simulink model "Delfin"  (R2018b)
settings: Solver=VariableStepAuto  StartTime=0.0  StopTime=0.2  RelTol=1e-3
undefined symbols (not defined in the file): fn, L1b, R1b, Stv, U1, U2, Ukz
libraries: powerlib x34, peRmsMeasurement x10, powerlib_meascontrol x2
settings Model: Creator=sr1  LastModifiedBy=sr1

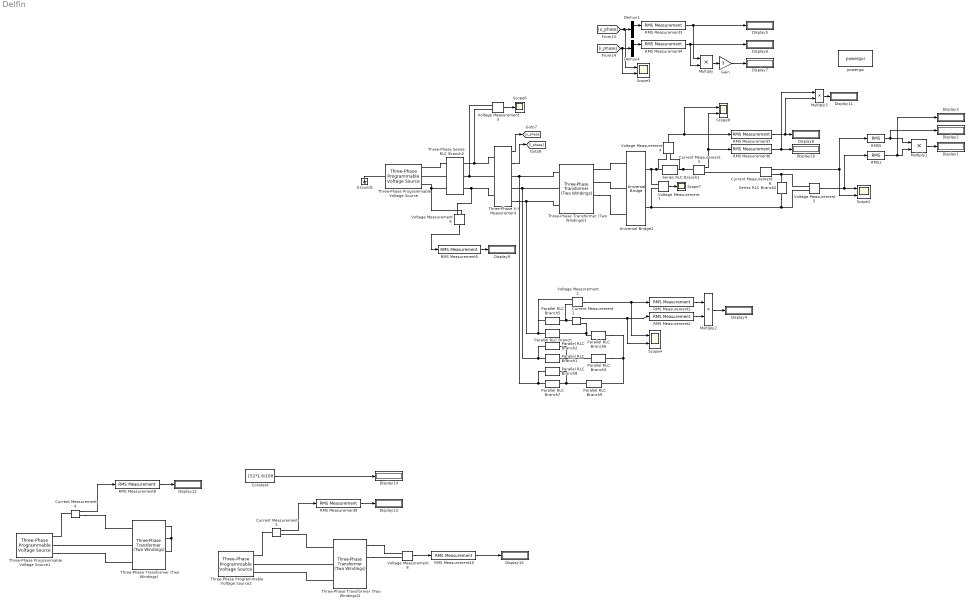
== system Delfin ==
  Constant : Constant  Value=152*1.6/100
  Current Measurement{1,3..6} (5 alike) : powerlib/Measurements/Current Measurement  PhasorSimulation=off  OutputType=Complex  PSBequivalent=0
  Demux1 : Demux  Outputs=3
  Demux4 : Demux  Outputs=3
  Display{1..15} (15 alike) : Display
  Gain : Gain  Gain=3
  Ground1 : powerlib/Elements/Ground  LConnTagsString=a
  Multiply{,1..3} (4 alike) : Product
  Parallel RLC Branch : powerlib/Elements/Parallel RLC Branch  LConnTagsString=a  RConnTagsString=__new0  BranchType=R  Resistance=680000  Inductance=1e-3  SetiL0=off  InitialCurrent=0  Capacitance=4e-6  Setx0=off  InitialVoltage=0  Measurements=None
  Parallel RLC Branch1 : powerlib/Elements/Parallel RLC Branch  LConnTagsString=a  RConnTagsString=__new0  BranchType=R  Resistance=680000  Inductance=1e-3  SetiL0=off  InitialCurrent=0  Capacitance=4e-6  Setx0=off  InitialVoltage=0  Measurements=None
  Parallel RLC Branch2 : powerlib/Elements/Parallel RLC Branch  LConnTagsString=a  RConnTagsString=__new0  BranchType=C  Resistance=47  Inductance=1e-3  SetiL0=off  InitialCurrent=0  Capacitance=4e-6  Setx0=off  InitialVoltage=0  Measurements=None
  Parallel RLC Branch3 : powerlib/Elements/Parallel RLC Branch  LConnTagsString=a  RConnTagsString=__new0  BranchType=R  Resistance=0.0001  Inductance=1e-3  SetiL0=off  InitialCurrent=0  Capacitance=4e-6  Setx0=off  InitialVoltage=0  Measurements=None
  Parallel RLC Branch5 : powerlib/Elements/Parallel RLC Branch  LConnTagsString=a  RConnTagsString=__new0  BranchType=C  Resistance=47  Inductance=1e-3  SetiL0=off  InitialCurrent=0  Capacitance=4e-6  Setx0=off  InitialVoltage=0  Measurements=None
  Parallel RLC Branch6 : powerlib/Elements/Parallel RLC Branch  LConnTagsString=a  RConnTagsString=__new0  BranchType=R  Resistance=0.0001  Inductance=1e-3  SetiL0=off  InitialCurrent=0  Capacitance=4e-6  Setx0=off  InitialVoltage=0  Measurements=None
  Parallel RLC Branch7 : powerlib/Elements/Parallel RLC Branch  LConnTagsString=a  RConnTagsString=__new0  BranchType=R  Resistance=680000  Inductance=1e-3  SetiL0=off  InitialCurrent=0  Capacitance=4e-6  Setx0=off  InitialVoltage=0  Measurements=None
  Parallel RLC Branch8 : powerlib/Elements/Parallel RLC Branch  LConnTagsString=a  RConnTagsString=__new0  BranchType=C  Resistance=47  Inductance=1e-3  SetiL0=off  InitialCurrent=0  Capacitance=4e-6  Setx0=off  InitialVoltage=0  Measurements=None
  Parallel RLC Branch9 : powerlib/Elements/Parallel RLC Branch  LConnTagsString=a  RConnTagsString=__new0  BranchType=R  Resistance=0.0001  Inductance=1e-3  SetiL0=off  InitialCurrent=0  Capacitance=4e-6  Setx0=off  InitialVoltage=0  Measurements=None
  RMS Measurement{1..2,8..10} (5 alike) : peRmsMeasurement/RMS Measurement  LabelModeActiveChoice=Harmonic  F=50  SpecifyHarmonics=on  K=[1 5 7 11 13]  Ts=0
  RMS Measurement3 : peRmsMeasurement/RMS Measurement  LabelModeActiveChoice=Harmonic  F=50  SpecifyHarmonics=on  K=[1]  Ts=0
  RMS Measurement4 : peRmsMeasurement/RMS Measurement  LabelModeActiveChoice=Harmonic  F=50  SpecifyHarmonics=on  K=[1]  Ts=0
  RMS Measurement5 : peRmsMeasurement/RMS Measurement  LabelModeActiveChoice=Harmonic  F=50  SpecifyHarmonics=on  K=[1]  Ts=0
  RMS Measurement6 : peRmsMeasurement/RMS Measurement  LabelModeActiveChoice=Harmonic  F=300  SpecifyHarmonics=on  K=[1 2 3 4 5]  Ts=0
  RMS Measurement7 : peRmsMeasurement/RMS Measurement  LabelModeActiveChoice=Harmonic  F=300  SpecifyHarmonics=on  K=[1 2 3 4 5]  Ts=0
  RMS1 : powerlib_meascontrol/Measurements/RMS  TrueRMS=on  Freq=300  RMSInit=0  Ts=0
  RMS5 : powerlib_meascontrol/Measurements/RMS  TrueRMS=on  Freq=300  RMSInit=0  Ts=0
  Scope{1,3..4,8} (4 alike) : Scope  NumInputPorts=2
  Scope6 : Scope
  Scope7 : Scope
  Series RLC Branch1 : powerlib/Elements/Series RLC Branch  LConnTagsString=__new0  RConnTagsString=__new0  BranchType=RL  Resistance=0.0001  Inductance=1.5e-3  SetiL0=off  InitialCurrent=0  Capacitance=5e-7  Setx0=off  InitialVoltage=0  Measurements=None
  Series RLC Branch2 : powerlib/Elements/Series RLC Branch  LConnTagsString=__new0  RConnTagsString=__new0  BranchType=R  Resistance=0.57  Inductance=250e-6  SetiL0=off  InitialCurrent=0  Capacitance=5e-7  Setx0=off  InitialVoltage=0  Measurements=None
  Three-Phase Programmable Voltage Source : powerlib/Electrical Sources/Three-Phase Programmable Voltage Source  PositiveSequence=[380 0 50]  VariationEntity=None  VariationType=Table of time-amplitude pairs  VariationTypeAlt=Step  VariationStep=0.5  VariationRate=10  VariationMagnitude=0.3  VariationFrequency=2  VariationTiming=[1 2]  VariationPhaseA=off  Amplitudes=[1 0.8 1.2 1.0]  TimeValues=[0 0.1 0.15 0.2]  HarmonicGeneration=off  HarmonicA=[3 0.2 -25 0]  HarmonicB=[2 0.15 35 2]  Timing="[0.05  3]"  BusType=swing  Pref=0  Qref=0  Qmin=-inf  Qmax=inf
  Three-Phase Programmable Voltage Source1 : powerlib/Electrical Sources/Three-Phase Programmable Voltage Source  PositiveSequence=[U1*(Ukz/100) 0 50]  VariationEntity=None  VariationType=Table of time-amplitude pairs  VariationTypeAlt=Step  VariationStep=0.5  VariationRate=10  VariationMagnitude=0.3  VariationFrequency=2  VariationTiming=[1 2]  VariationPhaseA=off  Amplitudes=[1 0.8 1.2 1.0]  TimeValues=[0 0.1 0.15 0.2]  HarmonicGeneration=off  HarmonicA=[3 0.2 -25 0]  HarmonicB=[2 0.15 35 2]  Timing="[0.05  3]"  BusType=swing  Pref=0  Qref=0  Qmin=-inf  Qmax=inf
  Three-Phase Programmable Voltage Source2 : powerlib/Electrical Sources/Three-Phase Programmable Voltage Source  PositiveSequence=[U1 0 50]  VariationEntity=None  VariationType=Table of time-amplitude pairs  VariationTypeAlt=Step  VariationStep=0.5  VariationRate=10  VariationMagnitude=0.3  VariationFrequency=2  VariationTiming=[1 2]  VariationPhaseA=off  Amplitudes=[1 0.8 1.2 1.0]  TimeValues=[0 0.1 0.15 0.2]  HarmonicGeneration=off  HarmonicA=[3 0.2 -25 0]  HarmonicB=[2 0.15 35 2]  Timing="[0.05  3]"  BusType=swing  Pref=0  Qref=0  Qmin=-inf  Qmax=inf
  Three-Phase Series RLC Branch2 : powerlib/Elements/Three-Phase Series RLC Branch  LConnTagsString=A|B|C  RConnTagsString=A|B|C  BranchType=R  Resistance=0.03  Inductance=0.08  Capacitance=1e-6  Measurements=None
  Three-Phase Transformer (Two Windings) : powerlib/Elements/Three-Phase Transformer (Two Windings)  Winding1Connection=Y  Winding2Connection=Yn  CoreType=Three single-phase transformers  SetSaturation=off  Hysteresis=off  DataFile='hysteresis'  SetInitialFlux=off  Measurements=None  UNITS=pu  NominalPower=[ Stv , fn ]  Winding1=[U1, R1b, L1b]  Winding2=[U2, R1b, L1b]  Rm=Ru  Lm=Lu  L0=0.5  Saturation=[0 0;0.0024 1.2;1 1.52]  InitialFluxes=[0.8 -0.8 0.69999]  MoreParameters=off  BreakLoop=off  DataType=off  TransfoNumber=1
  Three-Phase Transformer (Two Windings)1 : powerlib/Elements/Three-Phase Transformer (Two Windings)  Winding1Connection=Y  Winding2Connection=Yn  CoreType=Three single-phase transformers  SetSaturation=off  Hysteresis=off  DataFile='hysteresis'  SetInitialFlux=off  Measurements=None  UNITS=pu  NominalPower=[ Stv , fn ]  Winding1=[U1, R1b, L1b]  Winding2=[U2, R1b, L1b]  Rm=Ru  Lm=Lu  L0=0.5  Saturation=[0 0;0.0024 1.2;1 1.52]  InitialFluxes=[0.8 -0.8 0.69999]  MoreParameters=off  BreakLoop=off  DataType=off  TransfoNumber=1
  Three-Phase Transformer (Two Windings)2 : powerlib/Elements/Three-Phase Transformer (Two Windings)  Winding1Connection=Y  Winding2Connection=Yn  CoreType=Three single-phase transformers  SetSaturation=off  Hysteresis=off  DataFile='hysteresis'  SetInitialFlux=off  Measurements=None  UNITS=pu  NominalPower=[ Stv , fn ]  Winding1=[U1, R1b, L1b]  Winding2=[U2, R1b, L1b]  Rm=Ru  Lm=Lu  L0=0.5  Saturation=[0 0;0.0024 1.2;1 1.52]  InitialFluxes=[0.8 -0.8 0.69999]  MoreParameters=off  BreakLoop=off  DataType=off  TransfoNumber=1
  Three-Phase V-I Measurement : powerlib/Measurements/Three-Phase V-I Measurement  VoltageMeasurement=phase-to-ground  SetLabelV=off  LabelV=Vabc  Vpu=off  VpuLL=off  CurrentMeasurement=yes  SetLabelI=off  LabelI=Iabc  Ipu=off  Pbase=100e6  Vbase=500e3  OutputType=Complex  PhasorSimulation=off  PSBequivalent=0
  Universal Bridge1 : powerlib/Power Electronics/Universal Bridge  Arms=3  SnubberResistance=10  SnubberCapacitance=5e-7  Device=Diodes  Ron=380e-6  Lon=0  ForwardVoltages="[  0  0  ]"  ForwardVoltage=1  GTOparameters=[ 10e-6 , 20e-6 ]  IGBTparameters=[ 1e-6 , 2e-6 ]  Measurements=None  Measurements_2=None  converterType=Rectifier
  Voltage Measurement{2..8} (7 alike) : powerlib/Measurements/Voltage Measurement  PhasorSimulation=off  OutputType=Complex  PSBequivalent=0
  powergui : powerlib/powergui  Priority=1  SimulationMode=Discrete  SampleTime=1e-6  frequency=60  Iterations=50  frequencyindice=50  Pbase=100e6  ErrMax=1e-4  UnitsV=kV  UnitsW=MW  buscounter=0  FunctionMessages=off  echomessages=off  EnableUseOfTLC=off  CurrentSourceSwitches=off  DisableSnubberDevices=off  DisableRonSwitches=off  DisableVfSwitches=off  DisplayEquations=off  SolverType=Tustin/Backward Euler (TBE)  Interpol=off  ExternalGateDelay=off  methode=off  Ts=100  x0status=blocks  SPID=on  SwTol=0  HookPort=off  RestoreLinks=warning  ResistiveCurrentMeasurement=off  Frange=[0:2:500]  Ylog=off  Xlog=on  ShowGrid=off  save=off  variable=ZData  structure=logsout  ZoomFFT=off  StartTime=0.04  cycles=8  DisplayStyle=1  fundamental=50  FreqAxis=off  MaxFrequency=12000  frequencyindicesteady=1  RmsSteady=1  display=off
  wires:
  Three-Phase V-I Measurement/1 -> [u_phase]
  Three-Phase V-I Measurement/2 -> [i_phase]
  Gain/1 -> Display7/1
  Demux1/1 -> RMS Measurement3/1
  RMS Measurement4/1 -> Display6/1, Multiply/2
  RMS Measurement3/1 -> Display5/1, Multiply/1
  [i_phase] -> Scope3/2, Demux4/1
  Multiply/1 -> Gain/1
  Demux4/1 -> RMS Measurement4/1
  [u_phase] -> Scope3/1, Demux1/1
  Current Measurement6/1 -> RMS5/1, Scope1/2
  Voltage Measurement5/1 -> RMS1/1, Scope1/1
  RMS5/1 -> Display2/1, Multiply1/1
  RMS1/1 -> Display3/1, Multiply1/2
  Multiply1/1 -> Display1/1
  Voltage Measurement2/1 -> RMS Measurement1/1, Scope4/1
  RMS Measurement1/1 -> Multiply2/1
  RMS Measurement2/1 -> Multiply2/2
  Multiply2/1 -> Display4/1
  Voltage Measurement3/1 -> Scope6/1
  Voltage Measurement4/1 -> Scope8/1, RMS Measurement7/1
  RMS Measurement7/1 -> Multiply3/2, Display8/1
  Voltage Measurement6/1 -> RMS Measurement5/1
  RMS Measurement5/1 -> Display9/1
  Current Measurement3/1 -> Scope8/2, RMS Measurement6/1
  RMS Measurement6/1 -> Display10/1, Multiply3/1
  Multiply3/1 -> Display11/1
  Voltage Measurement7/1 -> Scope7/1
  Current Measurement1/1 -> RMS Measurement2/1, Scope4/2
  Current Measurement4/1 -> RMS Measurement8/1
  RMS Measurement8/1 -> Display12/1
  Current Measurement5/1 -> RMS Measurement9/1
  RMS Measurement9/1 -> Display13/1
  Constant/1 -> Display14/1
  RMS Measurement10/1 -> Display15/1
  Voltage Measurement8/1 -> RMS Measurement10/1
  connections:
  Three-Phase Programmable Voltage Source/LConn1 -- Ground1/LConn1
  Three-Phase Series RLC Branch2/LConn2 -- Three-Phase Programmable Voltage Source/RConn2
  Voltage Measurement5/LConn1 -- Current Measurement6/RConn1 -- Series RLC Branch2/LConn1
  Parallel RLC Branch1/LConn1 -- Parallel RLC Branch2/LConn1 -- Three-Phase V-I Measurement/RConn2 -- Three-Phase Transformer (Two Windings)1/LConn2
  Three-Phase V-I Measurement/RConn3 -- Voltage Measurement2/LConn1 -- Parallel RLC Branch5/LConn1 -- Parallel RLC Branch/LConn1 -- Three-Phase Transformer (Two Windings)1/LConn3
  Series RLC Branch1/RConn1 -- Voltage Measurement7/LConn1 -- Universal Bridge1/RConn1 -- Voltage Measurement4/LConn1
  Series RLC Branch2/RConn1 -- Voltage Measurement7/LConn2 -- Universal Bridge1/RConn2 -- Voltage Measurement5/LConn2
  Current Measurement3/RConn1 -- Current Measurement6/LConn1
  Three-Phase Series RLC Branch2/LConn1 -- Three-Phase Programmable Voltage Source/RConn1
  Three-Phase Series RLC Branch2/LConn3 -- Voltage Measurement6/LConn1 -- Three-Phase Programmable Voltage Source/RConn3
  Three-Phase Series RLC Branch2/RConn2 -- Three-Phase V-I Measurement/LConn2 -- Voltage Measurement3/LConn1
  Three-Phase Series RLC Branch2/RConn3 -- Three-Phase V-I Measurement/LConn3 -- Voltage Measurement6/LConn2
  Three-Phase Series RLC Branch2/RConn1 -- Voltage Measurement3/LConn2 -- Three-Phase V-I Measurement/LConn1
  Current Measurement3/LConn1 -- Voltage Measurement4/LConn2 -- Series RLC Branch1/LConn1
  Parallel RLC Branch1/RConn1 -- Parallel RLC Branch3/LConn1 -- Parallel RLC Branch2/RConn1
  Parallel RLC Branch7/RConn1 -- Parallel RLC Branch9/LConn1 -- Parallel RLC Branch8/RConn1
  Three-Phase V-I Measurement/RConn1 -- Three-Phase Transformer (Two Windings)1/LConn1 -- Parallel RLC Branch8/LConn1 -- Parallel RLC Branch7/LConn1
  Parallel RLC Branch3/RConn1 -- Parallel RLC Branch9/RConn1 -- Parallel RLC Branch6/RConn1
  Parallel RLC Branch5/RConn1 -- Voltage Measurement2/LConn2 -- Current Measurement1/LConn1
  Current Measurement1/RConn1 -- Parallel RLC Branch/RConn1 -- Parallel RLC Branch6/LConn1
  Three-Phase Transformer (Two Windings)/RConn1 -- Three-Phase Transformer (Two Windings)/RConn3 -- Three-Phase Transformer (Two Windings)/RConn2
  Three-Phase Programmable Voltage Source1/RConn2 -- Three-Phase Transformer (Two Windings)/LConn2
  Three-Phase Programmable Voltage Source1/RConn3 -- Three-Phase Transformer (Two Windings)/LConn3
  Current Measurement4/LConn1 -- Three-Phase Programmable Voltage Source1/RConn1
  Current Measurement4/RConn1 -- Three-Phase Transformer (Two Windings)/LConn1
  Three-Phase Transformer (Two Windings)2/LConn3 -- Three-Phase Programmable Voltage Source2/RConn3
  Three-Phase Transformer (Two Windings)2/LConn2 -- Three-Phase Programmable Voltage Source2/RConn2
  Three-Phase Transformer (Two Windings)2/LConn1 -- Current Measurement5/RConn1
  Current Measurement5/LConn1 -- Three-Phase Programmable Voltage Source2/RConn1
  Three-Phase Transformer (Two Windings)2/RConn1 -- Voltage Measurement8/LConn1
  Three-Phase Transformer (Two Windings)2/RConn2 -- Voltage Measurement8/LConn2
  Three-Phase Transformer (Two Windings)1/RConn1 -- Universal Bridge1/LConn1
  Three-Phase Transformer (Two Windings)1/RConn2 -- Universal Bridge1/LConn2
  Three-Phase Transformer (Two Windings)1/RConn3 -- Universal Bridge1/LConn3
